simulink model "VehicleController"  (R2026b)
settings: Solver=ode45  StopTime=Simulation.StopTimeSmoke.Value
undefined symbols (not defined in the file): DefaultActuatorCommandBus, DefaultControllerDebugBus
settings Model: DataDictionary=VehicleData.sldd  Creator=Xu Dingyi  LastModifiedBy=29358

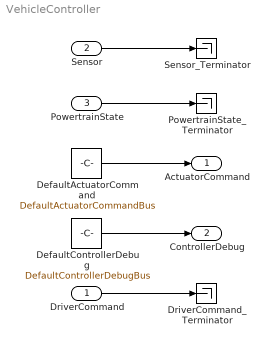
== system VehicleController ==
  DriverCommand : Inport  OutDataTypeStr=Bus: DriverCommandBus
  Sensor : Inport  Port=2  OutDataTypeStr=Bus: SensorBus
  PowertrainState : Inport  Port=3  OutDataTypeStr=Bus: PowertrainStateBus
  DefaultActuatorCommand : Constant  Value=DefaultActuatorCommandBus  OutDataTypeStr=Bus: ActuatorCommandBus  SampleTime=-1
  DefaultControllerDebug : Constant  Value=DefaultControllerDebugBus  OutDataTypeStr=Bus: ControllerDebugBus  SampleTime=-1
  DriverCommand_Terminator : Terminator
  PowertrainState_Terminator : Terminator
  Sensor_Terminator : Terminator
  ActuatorCommand : Outport  OutDataTypeStr=Bus: ActuatorCommandBus
  ControllerDebug : Outport  Port=2  OutDataTypeStr=Bus: ControllerDebugBus
  wires:
  DefaultControllerDebug/1 -> ControllerDebug/1
  DefaultActuatorCommand/1 -> ActuatorCommand/1
  PowertrainState/1 -> PowertrainState_Terminator/1
  Sensor/1 -> Sensor_Terminator/1
  DriverCommand/1 -> DriverCommand_Terminator/1
